simulink subsystem "Control_Velocidad"  (R2024b)
settings: Solver=VariableStepAuto  StartTime=0.0  StopTime=10.0  RelTol=1e-3
settings Model: Creator=Chenfu  LastModifiedBy=Chenfu

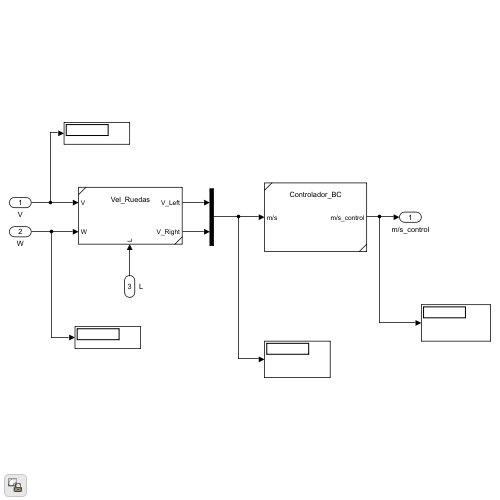
[thumbnail: Simulink's stored preview of the top-level diagram]
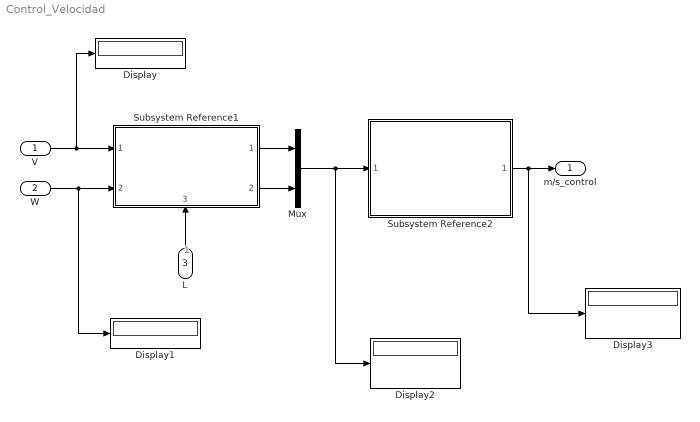
== system Control_Velocidad ==
  note: 1
  V : Inport
  W : Inport  Port=2
  L : Inport  Port=3
  Display{,1..3} (4 alike) : Display
  Mux : Mux  Inputs=2
  Subsystem Reference1 : Subsystem  ReferencedSubsystem=Vel_Ruedas
      settings: PortSchema="{\"entries\":[{\"content\":{\"sides\":[{\"content\":{\"connectorIds\":[\"In1\",\"In2\"]},\"type\":\"ConnectorPlacement.EquallySpacedRectSide\",\"uuid\":\"d84dcb5e-3d1f-491a-afee-794ad5554a2e\"},{\"content\":{\"connectorIds\":[\"Out1\",\"Out2\"],\"side\":\"RIGHT\"},\"type\":\"ConnectorPlacement.EquallySpacedRectSide\",\"uuid\":\"a0418b62-0e7f-41b6-9229-39e60bbbb316\"},{\"content\":{\"side\":\"TOP\"},\"type\":\"ConnectorPlacement.EquallySpacedRectSide\",\"uuid\":\"a2fa68ab-86c2-485e-93ce-d55ad9856492\"},{\"content\":{\"connectorIds\":[\"In3\"],\"side\":\"BOTTOM\"},\"type\":\"ConnectorPlacement.EquallySpacedRectSide\",\"uuid\":\"b1e52622-770d-4fba-ba7c-301b5de809e8\"}]},\"type\":\"ConnectorPlacement.EquallySpacedConnector\",\"uuid\":\"dfc2f15c-5eb1-4bff-a24d-1444b10fabc2\"}],\"packageUris\":[\"http://schema.mathworks.com/mf0/Connector/R2020b\"],\"version\":\"1.0\"}"
  Subsystem Reference2 : Subsystem  ReferencedSubsystem=Controlador_BC
  m/s_control : Outport
  wires:
  Mux/1 -> Subsystem Reference2/1, Display2/1
  Subsystem Reference1/1 -> Mux/1
  L/1 -> Subsystem Reference1/3
  Subsystem Reference1/2 -> Mux/2
  W/1 -> Subsystem Reference1/2, Display1/1
  V/1 -> Subsystem Reference1/1, Display/1
  Subsystem Reference2/1 -> m/s_control/1, Display3/1
